simulink model "Battery_Model"  (R2019b)
settings: configuration reference "BMS_Sw_CodeGenConfig" (kept outside this file)
undefined symbols (not defined in the file): Battery, TempInit, ts
libraries: BatteryPack_lib x37, fl_lib x5, nesl_utility x5
settings Model: DataDictionary=DD_Battery.sldd  EnableAccessToBaseWorkspace=off  Creator=mluethy  LastModifiedBy=cpatel
settings ConfigSetRef: SourceName=BMS_Sw_CodeGenConfig

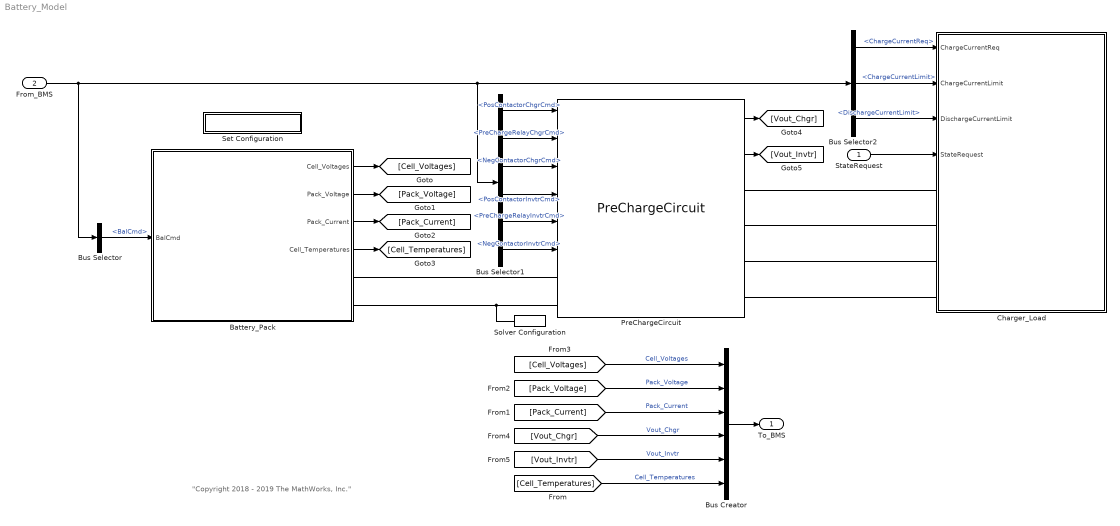
== system Battery_Model ==
  note: "Copyright 2018 - 2019 The MathWorks, Inc."
  StateRequest : Inport  OutDataTypeStr=Enum: SRE  SampleTime=[ts,0]  Interpolate=off
  From_BMS : Inport  Port=2  OutDataTypeStr=Bus: BMS_Output
  Battery_Pack : Subsystem  Variant=on  VariantControl=Variant1
      mask Display: image('Plant_Battery.jpg',[40,65,120,70])
  Bus Selector : BusSelector  OutputSignals=BalCmd
  Bus Selector1 : BusSelector  OutputSignals=PosContactorChgrCmd,PreChargeRelayChgrCmd,NegContactorChgrCmd,PosContactorInvtrCmd,PreChargeRelayInvtrCmd,NegContactorInvtrCmd
  Bus Selector2 : BusSelector  OutputSignals=ChargeCurrentReq,ChargeCurrentLimit,DischargeCurrentLimit
  Bus Creator : BusCreator  Inputs=6  OutDataTypeStr=Bus: BMS_Input  NonVirtualBus=on
  Charger_Load : Subsystem
      mask Display: image('Charger_Load3.jpg',[40,5,150,200])
  PreChargeCircuit : BatteryPack_lib/PreChargeCircuit  SystemSampleTime=-1  Latency=0  AutoFrameSizeCalculation=off
      mask Display: image('PowerElectronics.jpg',[110,60,100,100])
  Set Configuration : Subsystem
      mask Display: disp('Set Plant Configuration');
  Solver Configuration : nesl_utility/Solver Configuration  PhysicalDomain=network_engine_domain  SubClassName=solver  LeftPortType=input  RightPortType=generic  Tones=[]  Harmonics=[]  SimulateNoise=off  Profile=off  UseLocalSampling=off  EnableSwitchedLinearOptims=on  FrequencyDomain=off  UseCCode=off  RelTol=0.001  AbsTol=1e-06  MinStep=1e-09  ToWorkspace=off  RevertToSquareIcSolve=off  NumHomotopyIterations=100  PhasorMode=off  PhasorModeNumHarmonics=1  DoDC=off  ResidualTolerance=1e-09  UseLocalSolver=on  LocalSolverChoice=NE_BACKWARD_EULER_ADVANCER  LocalSolverSampleTime=ts  DoFixedCost=on  MaxNonlinIter=3  MaxModeIter=2  LinearAlgebra=auto  EquationFormulation=NE_TIME_EF  DelaysMemoryBudget=1024  AutomaticFiltering=on  FilteringTimeConstant=0.001  PartitionStorageMethod=AS_NEEDED  PartitionMemoryBudget=1024  PartitionMethod=FAST
  To_BMS : Outport  OutDataTypeStr=Bus: BMS_Input  VectorParamsAs1DForOutWhenUnconnected=off
  wires:
  Bus Selector1/2 -> PreChargeCircuit/2  "<PreChargeRelayChgrCmd>"
  Bus Selector1/3 -> PreChargeCircuit/3  "<NegContactorChgrCmd>"
  Bus Selector1/1 -> PreChargeCircuit/1  "<PosContactorChgrCmd>"
  Bus Selector1/4 -> PreChargeCircuit/4  "<PosContactorInvtrCmd>"
  Bus Selector1/6 -> PreChargeCircuit/6  "<NegContactorInvtrCmd>"
  Bus Selector1/5 -> PreChargeCircuit/5  "<PreChargeRelayInvtrCmd>"
  Bus Selector/1 -> Battery_Pack/1(BalCmd)  "<BalCmd>"
  From_BMS/1 -> Bus Selector1/1, Bus Selector2/1, Bus Selector/1
  Bus Selector2/1 -> Charger_Load/1(ChargeCurrentReq)  "<ChargeCurrentReq>"
  StateRequest/1 -> Charger_Load/4(StateRequest)
  Bus Creator/1 -> To_BMS/1
  Battery_Pack/1(Cell_Voltages) -> [Cell_Voltages]
  Battery_Pack/2(Pack_Voltage) -> [Pack_Voltage]
  Battery_Pack/3(Pack_Current) -> [Pack_Current]
  Battery_Pack/4(Cell_Temperatures) -> [Cell_Temperatures]
  [Cell_Voltages] -> Bus Creator/1  "Cell_Voltages"
  [Pack_Voltage] -> Bus Creator/2  "Pack_Voltage"
  [Pack_Current] -> Bus Creator/3  "Pack_Current"
  [Cell_Temperatures] -> Bus Creator/6  "Cell_Temperatures"
  PreChargeCircuit/1 -> [Vout_Chgr]
  PreChargeCircuit/2 -> [Vout_Invtr]
  [Vout_Chgr] -> Bus Creator/4  "Vout_Chgr"
  [Vout_Invtr] -> Bus Creator/5  "Vout_Invtr"
  Bus Selector2/2 -> Charger_Load/2(ChargeCurrentLimit)  "<ChargeCurrentLimit>"
  Bus Selector2/3 -> Charger_Load/3(DischargeCurrentLimit)  "<DischargeCurrentLimit>"
  connections:
  Solver Configuration/RConn1 -- Battery_Pack/RConn2 -- PreChargeCircuit/LConn2
  Battery_Pack/RConn1 -- PreChargeCircuit/LConn1
  PreChargeCircuit/RConn1 -- Charger_Load/LConn1
  PreChargeCircuit/RConn2 -- Charger_Load/LConn2
  Charger_Load/LConn3 -- PreChargeCircuit/RConn3
  Charger_Load/LConn4 -- PreChargeCircuit/RConn4

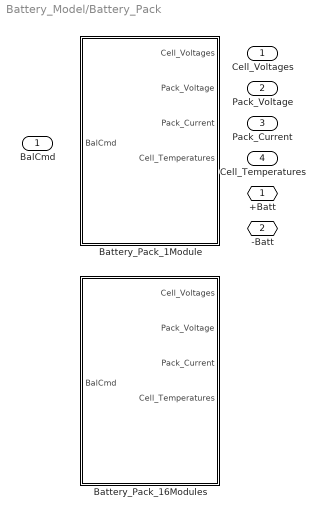
== system Battery_Model/Battery_Pack ==
  BalCmd : Inport
  Battery_Pack_16Modules : Subsystem  VariantControl=NumModules == 16
  Battery_Pack_1Module : Subsystem  VariantControl=NumModules == 1
  +Batt : PMIOPort  Side=Right
  -Batt : PMIOPort  Port=2  Side=Right
  Cell_Voltages : Outport  VectorParamsAs1DForOutWhenUnconnected=off
  Pack_Voltage : Outport  Port=2  VectorParamsAs1DForOutWhenUnconnected=off
  Pack_Current : Outport  Port=3  VectorParamsAs1DForOutWhenUnconnected=off
  Cell_Temperatures : Outport  Port=4  VectorParamsAs1DForOutWhenUnconnected=off

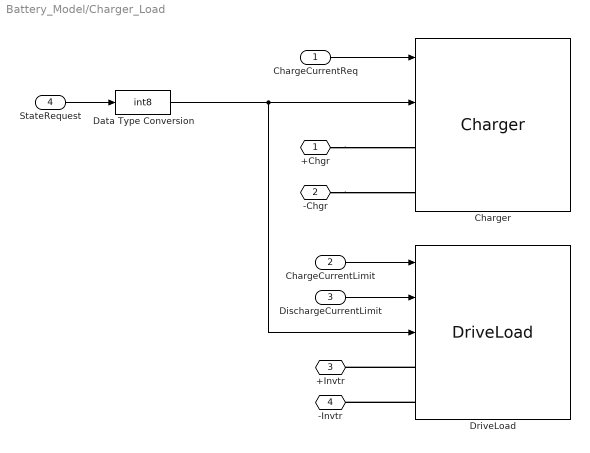
== system Battery_Model/Charger_Load ==
  ChargeCurrentReq : Inport
  ChargeCurrentLimit : Inport  Port=2
  DischargeCurrentLimit : Inport  Port=3
  StateRequest : Inport  Port=4
  Charger : BatteryPack_lib/Charger  SystemSampleTime=-1  Latency=0  AutoFrameSizeCalculation=off
      mask Display: image('Charger.jpg',[60,35,90,90])
  Data Type Conversion : DataTypeConversion  OutDataTypeStr=int8
  DriveLoad : BatteryPack_lib/DriveLoad  SystemSampleTime=-1  Latency=0  AutoFrameSizeCalculation=off
      mask Display: image('Load.jpg',[60,35,90,90])
  +Chgr : PMIOPort  Side=Left
  -Chgr : PMIOPort  Port=2  Side=Left
  +Invtr : PMIOPort  Port=3  Side=Left
  -Invtr : PMIOPort  Port=4  Side=Left
  wires:
  ChargeCurrentReq/1 -> Charger/1
  Data Type Conversion/1 -> DriveLoad/3, Charger/2
  StateRequest/1 -> Data Type Conversion/1
  DischargeCurrentLimit/1 -> DriveLoad/2
  ChargeCurrentLimit/1 -> DriveLoad/1
  connections:
  DriveLoad/LConn1 -- +Invtr/RConn1
  +Chgr/RConn1 -- Charger/LConn1
  DriveLoad/LConn2 -- -Invtr/RConn1
  -Chgr/RConn1 -- Charger/LConn2

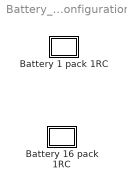
== system Battery_Model/Set Configuration ==
  Battery 1 pack 1RC : Subsystem
      settings: OpenFcn=|
      | SharedDictionaryObj = Simulink.data.dictionary.open('Shared_DD.sldd');
      | try removeDataSource(SharedDictionaryObj,'Battery_1Pack_1RC.sldd')
      | end
      | try removeDataSource(SharedDictionaryObj,'Battery_16Packs_1RC.sldd')
      | end
      | addDataSource(SharedDictionaryObj,'Battery_1Pack_1RC.sldd')
  Battery 16 pack 1RC : Subsystem
      settings: OpenFcn=|
      | SharedDictionaryObj = Simulink.data.dictionary.open('Shared_DD.sldd');
      | try removeDataSource(SharedDictionaryObj,'Battery_1Pack_1RC.sldd')
      | end
      | try removeDataSource(SharedDictionaryObj,'Battery_16Packs_1RC.sldd')
      | end
      | addDataSource(SharedDictionaryObj,'Battery_16Packs_1RC.sldd')

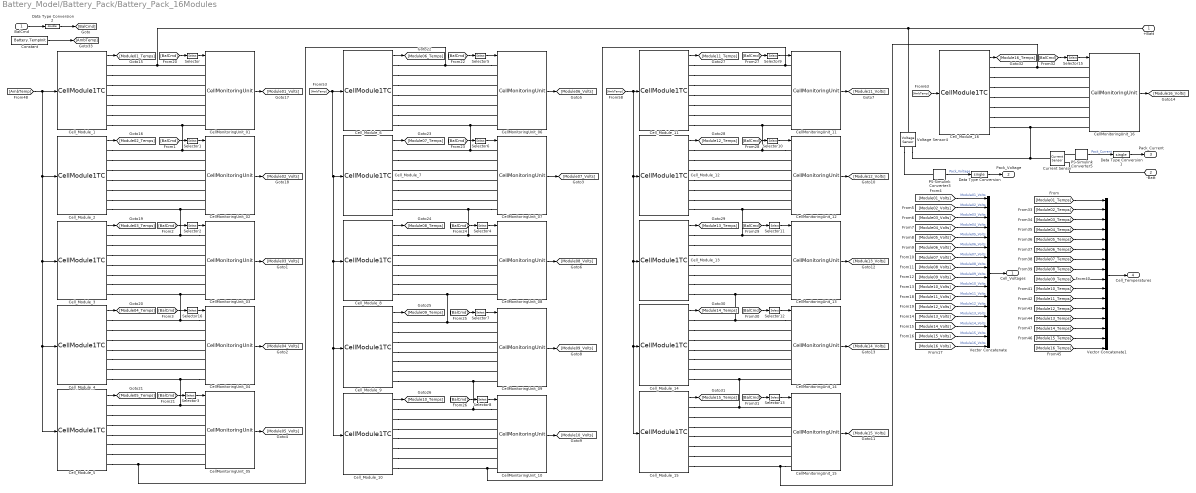
== system Battery_Model/Battery_Pack/Battery_Pack_16Modules ==
  BalCmd : Inport
  CellMonitoringUnit_01 : BatteryPack_lib/CellMonitoringUnit  SystemSampleTime=-1  Latency=0  AutoFrameSizeCalculation=off
  CellMonitoringUnit_02 : BatteryPack_lib/CellMonitoringUnit  SystemSampleTime=-1  Latency=0  AutoFrameSizeCalculation=off
  CellMonitoringUnit_03 : BatteryPack_lib/CellMonitoringUnit  SystemSampleTime=-1  Latency=0  AutoFrameSizeCalculation=off
  CellMonitoringUnit_04 : BatteryPack_lib/CellMonitoringUnit  SystemSampleTime=-1  Latency=0  AutoFrameSizeCalculation=off
  CellMonitoringUnit_05 : BatteryPack_lib/CellMonitoringUnit  SystemSampleTime=-1  Latency=0  AutoFrameSizeCalculation=off
  CellMonitoringUnit_06 : BatteryPack_lib/CellMonitoringUnit  SystemSampleTime=-1  Latency=0  AutoFrameSizeCalculation=off
  CellMonitoringUnit_07 : BatteryPack_lib/CellMonitoringUnit  SystemSampleTime=-1  Latency=0  AutoFrameSizeCalculation=off
  CellMonitoringUnit_08 : BatteryPack_lib/CellMonitoringUnit  SystemSampleTime=-1  Latency=0  AutoFrameSizeCalculation=off
  CellMonitoringUnit_09 : BatteryPack_lib/CellMonitoringUnit  SystemSampleTime=-1  Latency=0  AutoFrameSizeCalculation=off
  CellMonitoringUnit_{10..16} (7 alike) : BatteryPack_lib/CellMonitoringUnit  SystemSampleTime=-1  Latency=0  AutoFrameSizeCalculation=off
  Cell_Module_{1..16} (16 alike) : BatteryPack_lib/CellModule1TC  SystemSampleTime=-1  Latency=0  AutoFrameSizeCalculation=off
  Constant : Constant  Value=Battery.TempInit  SampleTime=ts
  Current Sensor : fl_lib/Electrical/Electrical Sensors/Current Sensor
  Data Type Conversion : DataTypeConversion  OutDataTypeStr=single
  Data Type Conversion1 : DataTypeConversion  OutDataTypeStr=single
  Data Type Conversion2 : DataTypeConversion  OutDataTypeStr=double
  PS-Simulink Converter3 : nesl_utility/PS-Simulink Converter  PhysicalDomain=network_engine_domain  SubClassName=ps_output  LeftPortType=input  RightPortType=output  PseudoPeriodic=off  Frequencies=[]  Unit=V  AffineConversion=off
  PS-Simulink Converter5 : nesl_utility/PS-Simulink Converter  PhysicalDomain=network_engine_domain  SubClassName=ps_output  LeftPortType=input  RightPortType=output  PseudoPeriodic=off  Frequencies=[]  Unit=A  AffineConversion=off
  Selector : Selector  InputPortWidth=96  IndexOptions=Starting index (dialog)  Indices=[1]  OutputSizes=6
  Selector1 : Selector  InputPortWidth=96  IndexOptions=Starting index (dialog)  Indices=7  OutputSizes=6
  Selector10 : Selector  InputPortWidth=96  IndexOptions=Starting index (dialog)  Indices=67  OutputSizes=6
  Selector11 : Selector  InputPortWidth=96  IndexOptions=Starting index (dialog)  Indices=73  OutputSizes=6
  Selector12 : Selector  InputPortWidth=96  IndexOptions=Starting index (dialog)  Indices=79  OutputSizes=6
  Selector13 : Selector  InputPortWidth=96  IndexOptions=Starting index (dialog)  Indices=85  OutputSizes=6
  Selector15 : Selector  InputPortWidth=96  IndexOptions=Starting index (dialog)  Indices=16  OutputSizes=6
  Selector16 : Selector  InputPortWidth=96  IndexOptions=Starting index (dialog)  Indices=19  OutputSizes=6
  Selector2 : Selector  InputPortWidth=96  IndexOptions=Starting index (dialog)  Indices=13  OutputSizes=6
  Selector3 : Selector  InputPortWidth=96  IndexOptions=Starting index (dialog)  Indices=25  OutputSizes=6
  Selector4 : Selector  InputPortWidth=96  IndexOptions=Starting index (dialog)  Indices=43  OutputSizes=6
  Selector5 : Selector  InputPortWidth=96  IndexOptions=Starting index (dialog)  Indices=31  OutputSizes=6
  Selector6 : Selector  InputPortWidth=96  IndexOptions=Starting index (dialog)  Indices=37  OutputSizes=6
  Selector7 : Selector  InputPortWidth=96  IndexOptions=Starting index (dialog)  Indices=49  OutputSizes=6
  Selector8 : Selector  InputPortWidth=96  IndexOptions=Starting index (dialog)  Indices=55  OutputSizes=6
  Selector9 : Selector  InputPortWidth=96  IndexOptions=Starting index (dialog)  Indices=61  OutputSizes=6
  Vector Concatenate : Concatenate  NumInputs=16
  Vector Concatenate1 : Concatenate  NumInputs=16
  Voltage Sensor4 : fl_lib/Electrical/Electrical Sensors/Voltage Sensor
  +Batt : PMIOPort  Side=Right
  -Batt : PMIOPort  Port=2  Side=Right
  Cell_Voltages : Outport  VectorParamsAs1DForOutWhenUnconnected=off
  Pack_Voltage : Outport  Port=2  VectorParamsAs1DForOutWhenUnconnected=off
  Pack_Current : Outport  Port=3  VectorParamsAs1DForOutWhenUnconnected=off
  Cell_Temperatures : Outport  Port=4  VectorParamsAs1DForOutWhenUnconnected=off
  wires:
  BalCmd/1 -> Data Type Conversion2/1
  Data Type Conversion2/1 -> [BalCmd]
  PS-Simulink Converter3/1 -> Data Type Conversion/1  "Pack_Voltage"
  PS-Simulink Converter5/1 -> Data Type Conversion1/1  "Pack_Current"
  [Module01_Volts] -> Vector Concatenate/1  "Module01_Volts"
  Vector Concatenate/1 -> Cell_Voltages/1
  [Module02_Volts] -> Vector Concatenate/2  "Module02_Volts"
  [Module03_Volts] -> Vector Concatenate/3  "Module03_Volts"
  [Module04_Volts] -> Vector Concatenate/4  "Module04_Volts"
  [Module05_Volts] -> Vector Concatenate/5  "Module05_Volts"
  [Module10_Volts] -> Vector Concatenate/10  "Module10_Volts"
  [Module09_Volts] -> Vector Concatenate/9  "Module09_Volts"
  [Module08_Volts] -> Vector Concatenate/8  "Module08_Volts"
  [Module07_Volts] -> Vector Concatenate/7  "Module07_Volts"
  [Module06_Volts] -> Vector Concatenate/6  "Module06_Volts"
  [Module11_Volts] -> Vector Concatenate/11  "Module11_Volts"
  [Module12_Volts] -> Vector Concatenate/12  "Module12_Volts"
  [Module13_Volts] -> Vector Concatenate/13  "Module13_Volts"
  [Module14_Volts] -> Vector Concatenate/14  "Module14_Volts"
  [Module15_Volts] -> Vector Concatenate/15  "Module15_Volts"
  [Module16_Volts] -> Vector Concatenate/16  "Module16_Volts"
  [BalCmd] -> Selector/1
  CellMonitoringUnit_01/1 -> [Module01_Volts]
  CellMonitoringUnit_02/1 -> [Module02_Volts]
  Selector16/1 -> CellMonitoringUnit_04/1
  CellMonitoringUnit_04/1 -> [Module04_Volts]
  CellMonitoringUnit_03/1 -> [Module03_Volts]
  Selector2/1 -> CellMonitoringUnit_03/1
  CellMonitoringUnit_08/1 -> [Module08_Volts]
  Selector4/1 -> CellMonitoringUnit_08/1
  CellMonitoringUnit_06/1 -> [Module06_Volts]
  Selector5/1 -> CellMonitoringUnit_06/1
  Selector6/1 -> CellMonitoringUnit_07/1
  Selector3/1 -> CellMonitoringUnit_05/1
  CellMonitoringUnit_07/1 -> [Module07_Volts]
  CellMonitoringUnit_05/1 -> [Module05_Volts]
  CellMonitoringUnit_12/1 -> [Module12_Volts]
  CellMonitoringUnit_10/1 -> [Module10_Volts]
  CellMonitoringUnit_09/1 -> [Module09_Volts]
  Selector7/1 -> CellMonitoringUnit_09/1
  CellMonitoringUnit_11/1 -> [Module11_Volts]
  CellMonitoringUnit_16/1 -> [Module16_Volts]
  CellMonitoringUnit_14/1 -> [Module14_Volts]
  CellMonitoringUnit_13/1 -> [Module13_Volts]
  CellMonitoringUnit_15/1 -> [Module15_Volts]
  Selector/1 -> CellMonitoringUnit_01/1
  [BalCmd] -> Selector1/1
  [BalCmd] -> Selector2/1
  [BalCmd] -> Selector16/1
  [BalCmd] -> Selector3/1
  [BalCmd] -> Selector5/1
  [BalCmd] -> Selector6/1
  [BalCmd] -> Selector4/1
  [BalCmd] -> Selector7/1
  [BalCmd] -> Selector8/1
  Selector8/1 -> CellMonitoringUnit_10/1
  [BalCmd] -> Selector9/1
  Selector9/1 -> CellMonitoringUnit_11/1
  [BalCmd] -> Selector10/1
  Selector10/1 -> CellMonitoringUnit_12/1
  [BalCmd] -> Selector11/1
  Selector11/1 -> CellMonitoringUnit_13/1
  [BalCmd] -> Selector12/1
  Selector12/1 -> CellMonitoringUnit_14/1
  [BalCmd] -> Selector13/1
  Selector13/1 -> CellMonitoringUnit_15/1
  [BalCmd] -> Selector15/1
  Selector15/1 -> CellMonitoringUnit_16/1
  Data Type Conversion/1 -> Pack_Voltage/1
  Data Type Conversion1/1 -> Pack_Current/1
  Cell_Module_1/1 -> [Module01_Temps]
  Cell_Module_16/1 -> [Module16_Temps]
  [Module01_Temps] -> Vector Concatenate1/1
  [Module02_Temps] -> Vector Concatenate1/2
  [Module03_Temps] -> Vector Concatenate1/3
  [Module04_Temps] -> Vector Concatenate1/4
  [Module05_Temps] -> Vector Concatenate1/5
  [Module06_Temps] -> Vector Concatenate1/6
  [Module07_Temps] -> Vector Concatenate1/7
  [Module08_Temps] -> Vector Concatenate1/8
  [Module09_Temps] -> Vector Concatenate1/9
  [Module10_Temps] -> Vector Concatenate1/10
  [Module11_Temps] -> Vector Concatenate1/11
  [Module12_Temps] -> Vector Concatenate1/12
  [Module13_Temps] -> Vector Concatenate1/13
  [Module16_Temps] -> Vector Concatenate1/16
  [Module14_Temps] -> Vector Concatenate1/14
  [Module15_Temps] -> Vector Concatenate1/15
  Vector Concatenate1/1 -> Cell_Temperatures/1
  [AmbTemp] -> Cell_Module_1/1, Cell_Module_2/1, Cell_Module_3/1, Cell_Module_5/1, Cell_Module_4/1
  Constant/1 -> [AmbTemp]
  [AmbTemp] -> Cell_Module_16/1
  Selector1/1 -> CellMonitoringUnit_02/1
  Cell_Module_2/1 -> [Module02_Temps]
  Cell_Module_3/1 -> [Module03_Temps]
  Cell_Module_4/1 -> [Module04_Temps]
  Cell_Module_5/1 -> [Module05_Temps]
  [AmbTemp] -> Cell_Module_6/1, Cell_Module_7/1, Cell_Module_8/1, Cell_Module_10/1, Cell_Module_9/1
  Cell_Module_6/1 -> [Module06_Temps]
  Cell_Module_8/1 -> [Module08_Temps]
  Cell_Module_7/1 -> [Module07_Temps]
  Cell_Module_10/1 -> [Module10_Temps]
  Cell_Module_9/1 -> [Module09_Temps]
  Cell_Module_11/1 -> [Module11_Temps]
  Cell_Module_12/1 -> [Module12_Temps]
  Cell_Module_13/1 -> [Module13_Temps]
  Cell_Module_15/1 -> [Module15_Temps]
  Cell_Module_14/1 -> [Module14_Temps]
  [AmbTemp] -> Cell_Module_11/1, Cell_Module_12/1, Cell_Module_13/1, Cell_Module_14/1, Cell_Module_15/1
  connections:
  Cell_Module_1/RConn1 -- CellMonitoringUnit_01/LConn1 -- +Batt/RConn1 -- Voltage Sensor4/LConn1
  -Batt/RConn1 -- Current Sensor/RConn2
  Voltage Sensor4/RConn1 -- PS-Simulink Converter3/LConn1
  PS-Simulink Converter5/LConn1 -- Current Sensor/RConn1
  Cell_Module_1/RConn2 -- CellMonitoringUnit_01/LConn2
  Cell_Module_1/RConn3 -- CellMonitoringUnit_01/LConn3
  Cell_Module_1/RConn4 -- CellMonitoringUnit_01/LConn4
  Cell_Module_1/RConn5 -- CellMonitoringUnit_01/LConn5
  Cell_Module_1/RConn6 -- CellMonitoringUnit_01/LConn6
  Cell_Module_2/RConn5 -- CellMonitoringUnit_02/LConn5
  Cell_Module_2/RConn2 -- CellMonitoringUnit_02/LConn2
  Cell_Module_1/RConn7 -- CellMonitoringUnit_01/LConn7 -- Cell_Module_2/RConn1 -- CellMonitoringUnit_02/LConn1
  Cell_Module_2/RConn4 -- CellMonitoringUnit_02/LConn4
  Cell_Module_2/RConn3 -- CellMonitoringUnit_02/LConn3
  Cell_Module_2/RConn6 -- CellMonitoringUnit_02/LConn6
  CellMonitoringUnit_04/LConn1 -- Cell_Module_4/RConn1 -- Cell_Module_3/RConn7 -- CellMonitoringUnit_03/LConn7
  Cell_Module_4/RConn6 -- CellMonitoringUnit_04/LConn6
  Cell_Module_4/RConn3 -- CellMonitoringUnit_04/LConn3
  Cell_Module_4/RConn2 -- CellMonitoringUnit_04/LConn2
  Cell_Module_4/RConn4 -- CellMonitoringUnit_04/LConn4
  Cell_Module_4/RConn5 -- CellMonitoringUnit_04/LConn5
  Cell_Module_3/RConn6 -- CellMonitoringUnit_03/LConn6
  Cell_Module_3/RConn3 -- CellMonitoringUnit_03/LConn3
  Cell_Module_3/RConn4 -- CellMonitoringUnit_03/LConn4
  CellMonitoringUnit_03/LConn1 -- Cell_Module_3/RConn1 -- Cell_Module_2/RConn7 -- CellMonitoringUnit_02/LConn7
  Cell_Module_3/RConn5 -- CellMonitoringUnit_03/LConn5
  Cell_Module_3/RConn2 -- CellMonitoringUnit_03/LConn2
  CellMonitoringUnit_06/LConn1 -- Cell_Module_6/RConn1 -- Cell_Module_5/RConn7 -- CellMonitoringUnit_05/LConn7
  CellMonitoringUnit_07/LConn7 -- Cell_Module_7/RConn7 -- Cell_Module_8/RConn1 -- CellMonitoringUnit_08/LConn1
  Cell_Module_6/RConn7 -- CellMonitoringUnit_06/LConn7 -- Cell_Module_7/RConn1 -- CellMonitoringUnit_07/LConn1
  Cell_Module_7/RConn2 -- CellMonitoringUnit_07/LConn2
  Cell_Module_8/RConn2 -- CellMonitoringUnit_08/LConn2
  Cell_Module_8/RConn5 -- CellMonitoringUnit_08/LConn5
  Cell_Module_7/RConn4 -- CellMonitoringUnit_07/LConn4
  Cell_Module_5/RConn5 -- CellMonitoringUnit_05/LConn5
  Cell_Module_7/RConn3 -- CellMonitoringUnit_07/LConn3
  Cell_Module_6/RConn3 -- CellMonitoringUnit_06/LConn3
  Cell_Module_5/RConn2 -- CellMonitoringUnit_05/LConn2
  Cell_Module_6/RConn4 -- CellMonitoringUnit_06/LConn4
  Cell_Module_6/RConn6 -- CellMonitoringUnit_06/LConn6
  CellMonitoringUnit_04/LConn7 -- Cell_Module_4/RConn7 -- Cell_Module_5/RConn1 -- CellMonitoringUnit_05/LConn1
  Cell_Module_8/RConn3 -- CellMonitoringUnit_08/LConn3
  Cell_Module_7/RConn6 -- CellMonitoringUnit_07/LConn6
  Cell_Module_6/RConn5 -- CellMonitoringUnit_06/LConn5
  Cell_Module_5/RConn6 -- CellMonitoringUnit_05/LConn6
  Cell_Module_5/RConn4 -- CellMonitoringUnit_05/LConn4
  Cell_Module_8/RConn6 -- CellMonitoringUnit_08/LConn6
  Cell_Module_5/RConn3 -- CellMonitoringUnit_05/LConn3
  Cell_Module_7/RConn5 -- CellMonitoringUnit_07/LConn5
  Cell_Module_6/RConn2 -- CellMonitoringUnit_06/LConn2
  Cell_Module_8/RConn4 -- CellMonitoringUnit_08/LConn4
  CellMonitoringUnit_12/LConn1 -- Cell_Module_11/RConn7 -- CellMonitoringUnit_11/LConn7 -- Cell_Module_12/RConn1
  CellMonitoringUnit_10/LConn1 -- Cell_Module_10/RConn1 -- Cell_Module_9/RConn7 -- CellMonitoringUnit_09/LConn7
  Cell_Module_10/RConn7 -- CellMonitoringUnit_10/LConn7 -- Cell_Module_11/RConn1 -- CellMonitoringUnit_11/LConn1
  CellMonitoringUnit_08/LConn7 -- Cell_Module_8/RConn7 -- CellMonitoringUnit_09/LConn1 -- Cell_Module_9/RConn1
  Cell_Module_12/RConn6 -- CellMonitoringUnit_12/LConn6
  Cell_Module_9/RConn4 -- CellMonitoringUnit_09/LConn4
  Cell_Module_12/RConn2 -- CellMonitoringUnit_12/LConn2
  Cell_Module_9/RConn6 -- CellMonitoringUnit_09/LConn6
  Cell_Module_12/RConn3 -- CellMonitoringUnit_12/LConn3
  Cell_Module_10/RConn5 -- CellMonitoringUnit_10/LConn5
  Cell_Module_11/RConn4 -- CellMonitoringUnit_11/LConn4
  Cell_Module_9/RConn2 -- CellMonitoringUnit_09/LConn2
  Cell_Module_9/RConn3 -- CellMonitoringUnit_09/LConn3
  Cell_Module_13/RConn1 -- CellMonitoringUnit_13/LConn1 -- Cell_Module_12/RConn7 -- CellMonitoringUnit_12/LConn7
  Cell_Module_12/RConn5 -- CellMonitoringUnit_12/LConn5
  Cell_Module_10/RConn3 -- CellMonitoringUnit_10/LConn3
  Cell_Module_10/RConn6 -- CellMonitoringUnit_10/LConn6
  Cell_Module_10/RConn4 -- CellMonitoringUnit_10/LConn4
  Cell_Module_11/RConn6 -- CellMonitoringUnit_11/LConn6
  Cell_Module_11/RConn3 -- CellMonitoringUnit_11/LConn3
  Cell_Module_11/RConn2 -- CellMonitoringUnit_11/LConn2
  Cell_Module_10/RConn2 -- CellMonitoringUnit_10/LConn2
  Cell_Module_11/RConn5 -- CellMonitoringUnit_11/LConn5
  Cell_Module_12/RConn4 -- CellMonitoringUnit_12/LConn4
  Cell_Module_9/RConn5 -- CellMonitoringUnit_09/LConn5
  CellMonitoringUnit_14/LConn1 -- Cell_Module_13/RConn7 -- CellMonitoringUnit_13/LConn7 -- Cell_Module_14/RConn1
  CellMonitoringUnit_14/LConn7 -- Cell_Module_15/RConn1 -- CellMonitoringUnit_15/LConn1 -- Cell_Module_14/RConn7
  Cell_Module_16/RConn6 -- CellMonitoringUnit_16/LConn6
  Cell_Module_13/RConn4 -- CellMonitoringUnit_13/LConn4
  Cell_Module_16/RConn2 -- CellMonitoringUnit_16/LConn2
  Cell_Module_13/RConn6 -- CellMonitoringUnit_13/LConn6
  Cell_Module_16/RConn3 -- CellMonitoringUnit_16/LConn3
  Cell_Module_14/RConn5 -- CellMonitoringUnit_14/LConn5
  Cell_Module_15/RConn4 -- CellMonitoringUnit_15/LConn4
  Cell_Module_13/RConn2 -- CellMonitoringUnit_13/LConn2
  Cell_Module_13/RConn3 -- CellMonitoringUnit_13/LConn3
  Current Sensor/LConn1 -- Voltage Sensor4/RConn2 -- Cell_Module_16/RConn7 -- CellMonitoringUnit_16/LConn7
  Cell_Module_16/RConn5 -- CellMonitoringUnit_16/LConn5
  Cell_Module_14/RConn3 -- CellMonitoringUnit_14/LConn3
  Cell_Module_14/RConn6 -- CellMonitoringUnit_14/LConn6
  Cell_Module_14/RConn4 -- CellMonitoringUnit_14/LConn4
  Cell_Module_15/RConn6 -- CellMonitoringUnit_15/LConn6
  Cell_Module_15/RConn3 -- CellMonitoringUnit_15/LConn3
  Cell_Module_15/RConn2 -- CellMonitoringUnit_15/LConn2
  Cell_Module_14/RConn2 -- CellMonitoringUnit_14/LConn2
  Cell_Module_15/RConn5 -- CellMonitoringUnit_15/LConn5
  Cell_Module_16/RConn4 -- CellMonitoringUnit_16/LConn4
  Cell_Module_13/RConn5 -- CellMonitoringUnit_13/LConn5
  CellMonitoringUnit_15/LConn7 -- Cell_Module_15/RConn7 -- Cell_Module_16/RConn1 -- CellMonitoringUnit_16/LConn1

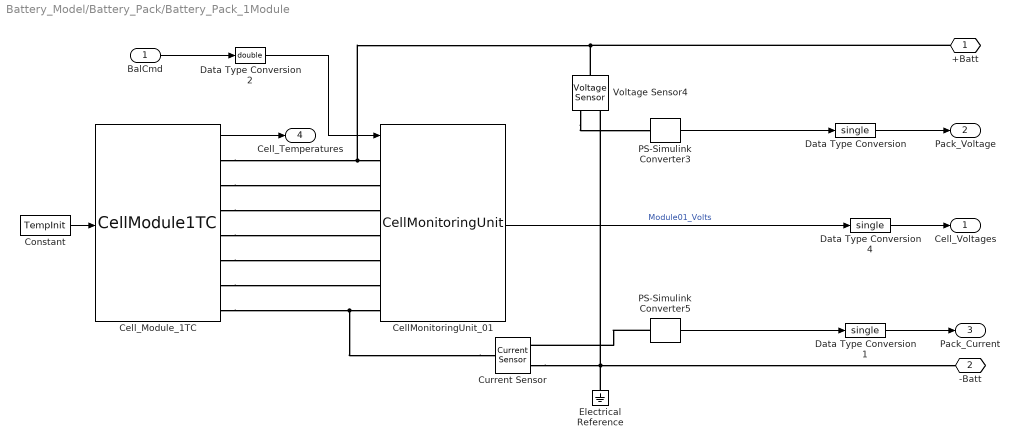
== system Battery_Model/Battery_Pack/Battery_Pack_1Module ==
  BalCmd : Inport
  CellMonitoringUnit_01 : BatteryPack_lib/CellMonitoringUnit  SystemSampleTime=-1  Latency=0  AutoFrameSizeCalculation=off
  Cell_Module_1TC : BatteryPack_lib/CellModule1TC  SystemSampleTime=-1  Latency=0  AutoFrameSizeCalculation=off
  Constant : Constant  Value=TempInit  SampleTime=ts
  Current Sensor : fl_lib/Electrical/Electrical Sensors/Current Sensor
  Data Type Conversion : DataTypeConversion  OutDataTypeStr=single
  Data Type Conversion1 : DataTypeConversion  OutDataTypeStr=single
  Data Type Conversion2 : DataTypeConversion  OutDataTypeStr=double
  Data Type Conversion4 : DataTypeConversion  OutDataTypeStr=single
  Electrical Reference : fl_lib/Electrical/Electrical Elements/Electrical Reference
  PS-Simulink Converter3 : nesl_utility/PS-Simulink Converter  PhysicalDomain=network_engine_domain  SubClassName=ps_output  LeftPortType=input  RightPortType=output  PseudoPeriodic=off  Frequencies=[]  Unit=V  AffineConversion=off
  PS-Simulink Converter5 : nesl_utility/PS-Simulink Converter  PhysicalDomain=network_engine_domain  SubClassName=ps_output  LeftPortType=input  RightPortType=output  PseudoPeriodic=off  Frequencies=[]  Unit=A  AffineConversion=off
  Voltage Sensor4 : fl_lib/Electrical/Electrical Sensors/Voltage Sensor
  +Batt : PMIOPort  Side=Right
  -Batt : PMIOPort  Port=2  Side=Right
  Cell_Voltages : Outport  VectorParamsAs1DForOutWhenUnconnected=off
  Pack_Voltage : Outport  Port=2  VectorParamsAs1DForOutWhenUnconnected=off
  Pack_Current : Outport  Port=3  VectorParamsAs1DForOutWhenUnconnected=off
  Cell_Temperatures : Outport  Port=4  VectorParamsAs1DForOutWhenUnconnected=off
  wires:
  BalCmd/1 -> Data Type Conversion2/1
  CellMonitoringUnit_01/1 -> Data Type Conversion4/1  "Module01_Volts"
  Data Type Conversion/1 -> Pack_Voltage/1
  Data Type Conversion1/1 -> Pack_Current/1
  Cell_Module_1TC/1 -> Cell_Temperatures/1
  PS-Simulink Converter5/1 -> Data Type Conversion1/1
  PS-Simulink Converter3/1 -> Data Type Conversion/1
  Data Type Conversion4/1 -> Cell_Voltages/1
  Constant/1 -> Cell_Module_1TC/1
  Data Type Conversion2/1 -> CellMonitoringUnit_01/1
  connections:
  +Batt/RConn1 -- Cell_Module_1TC/RConn1 -- CellMonitoringUnit_01/LConn1 -- Voltage Sensor4/LConn1
  Electrical Reference/LConn1 -- Current Sensor/RConn2 -- Voltage Sensor4/RConn2 -- -Batt/RConn1
  Voltage Sensor4/RConn1 -- PS-Simulink Converter3/LConn1
  PS-Simulink Converter5/LConn1 -- Current Sensor/RConn1
  Current Sensor/LConn1 -- Cell_Module_1TC/RConn7 -- CellMonitoringUnit_01/LConn7
  Cell_Module_1TC/RConn2 -- CellMonitoringUnit_01/LConn2
  Cell_Module_1TC/RConn3 -- CellMonitoringUnit_01/LConn3
  Cell_Module_1TC/RConn4 -- CellMonitoringUnit_01/LConn4
  Cell_Module_1TC/RConn5 -- CellMonitoringUnit_01/LConn5
  Cell_Module_1TC/RConn6 -- CellMonitoringUnit_01/LConn6

== system Battery_Model/Set Configuration/Battery 1 pack 1RC ==

== system Battery_Model/Set Configuration/Battery 16 pack 1RC ==
